simulink model "parte1_eje14_controlPD"  (R2017b)
settings: Solver=VariableStepAuto  StartTime=0.0  StopTime=20  RelTol=1e-3
libraries: simulink x1
settings Model: Creator=cjuar  LastModifiedBy=cjuar

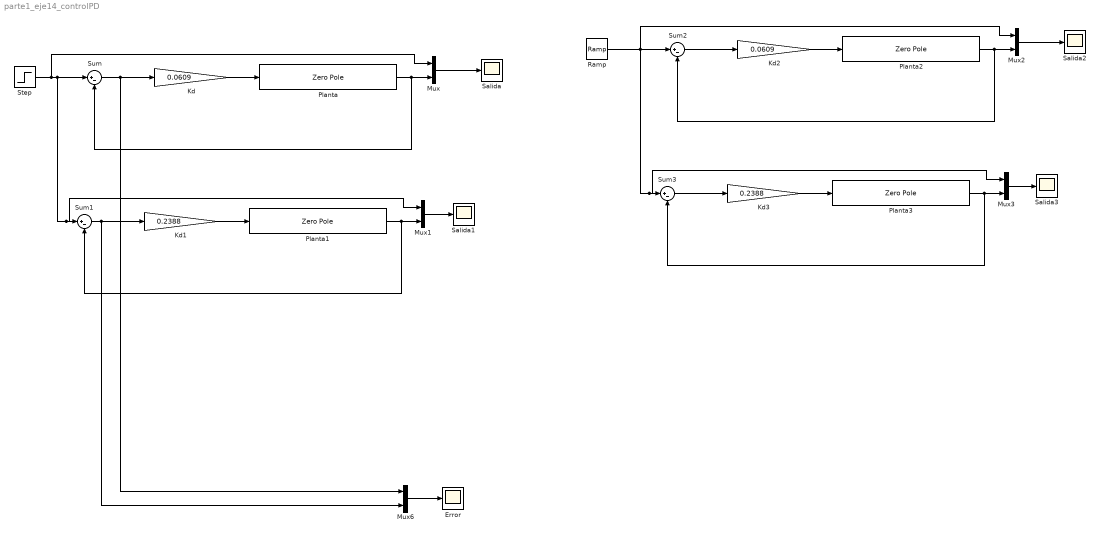
== system parte1_eje14_controlPD ==
  Error : Scope
  Kd : Gain  Gain=0.0609
  Kd1 : Gain  Gain=0.2388
  Kd2 : Gain  Gain=0.0609
  Kd3 : Gain  Gain=0.2388
  Mux{,1..3,6} (5 alike) : Mux  Inputs=2
  Planta : ZeroPole  Zeros=[-11.136]  Poles=[0 -6 -18]  Gain=1080
  Planta1 : ZeroPole  Zeros=[-4.4324]  Poles=[0 -6 -18]  Gain=1080
  Planta2 : ZeroPole  Zeros=[-11.136]  Poles=[0 -6 -18]  Gain=1080
  Planta3 : ZeroPole  Zeros=[-4.4324]  Poles=[0 -6 -18]  Gain=1080
  Ramp : simulink/Sources/Ramp  slope=1  start=0  X0=0
  Salida{,1..3} (4 alike) : Scope
  Step : Step  SampleTime=0
  Sum{,1..3} (4 alike) : Sum  Inputs=|+-
  wires:
  Sum/1 -> Mux6/1, Kd/1
  Planta/1 -> Sum/2, Mux/2
  Mux/1 -> Salida/1
  Mux6/1 -> Error/1
  Kd/1 -> Planta/1
  Kd1/1 -> Planta1/1
  Step/1 -> Mux/1, Mux1/1, Sum1/1, Sum/1
  Mux1/1 -> Salida1/1
  Planta1/1 -> Mux1/2, Sum1/2
  Sum1/1 -> Mux6/2, Kd1/1
  Sum3/1 -> Kd3/1
  Planta3/1 -> Sum3/2, Mux3/2
  Mux3/1 -> Salida3/1
  Ramp/1 -> Mux2/1, Sum2/1, Sum3/1, Mux3/1
  Kd3/1 -> Planta3/1
  Kd2/1 -> Planta2/1
  Mux2/1 -> Salida2/1
  Planta2/1 -> Mux2/2, Sum2/2
  Sum2/1 -> Kd2/1
